simulink model "fancy_dancy_racing_wheely"  (R2019b)
settings: Solver=VariableStepAuto  StartTime=0.0  StopTime=inf  RelTol=1e-3
libraries: dspsrcs4 x2
settings Model: EnablePacing=on  Creator=mandl  LastModifiedBy=mandl

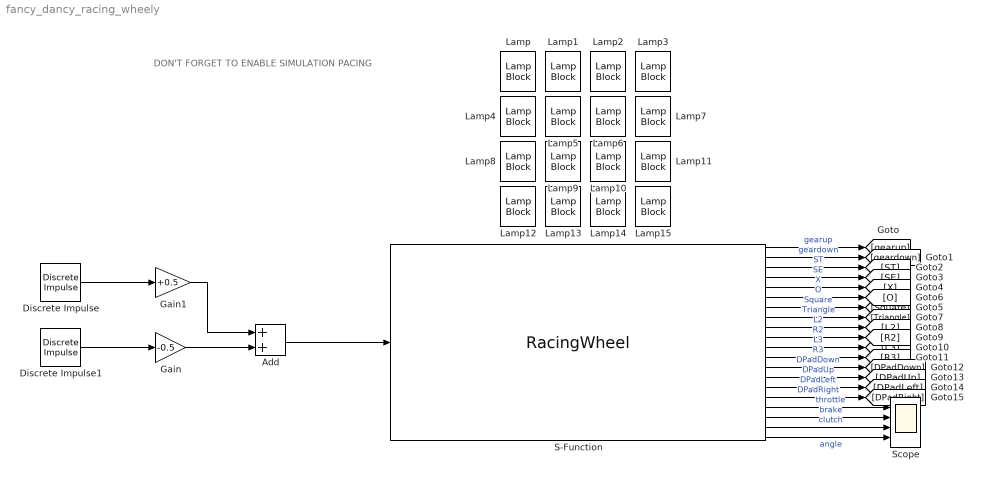
== system fancy_dancy_racing_wheely ==
  note: DON'T FORGET TO ENABLE SIMULATION PACING
  Add : Sum
  Discrete Impulse : dspsrcs4/Discrete  Impulse  Delay=500  SampleTime=0.01  FrameSample=1  OutputFrames=off  dataType=double  isSigned=on  wordLen=16  udDataType=sfix(16)  fracBitsMode=Best precision  numFracBits=15  OutDataTypeStr=double  LastOutDataTypeStr=double
  Discrete Impulse1 : dspsrcs4/Discrete  Impulse  Delay=1000  SampleTime=0.01  FrameSample=1  OutputFrames=off  dataType=double  isSigned=on  wordLen=16  udDataType=sfix(16)  fracBitsMode=Best precision  numFracBits=15  OutDataTypeStr=double  LastOutDataTypeStr=double
  Gain : Gain  Gain=-0.5
  Gain1 : Gain  Gain=+0.5
  Lamp{,1..15} (16 alike) : LampBlock
  S-Function : S-Function  FunctionName=RacingWheel  Parameters=Ts_FF uint32(1e5)  SFunctionModules=RacingWheel_wrapper  SFunctionDeploymentMode=off  EnableBusSupport=off  mask(Racing Wheel with Force Feedback){Ts_FF=0.01, Effect_duration=1e4}
      mask prompts: Ts_FF "Constant Force-Feedback Sample Time"; Effect_duration "Effect Duration in seconds (uint32)"
      mask help: Interacts with the windows gaming API from UWP. The force feedback effect is constant over the user defined sampling time below.
      mask init:
      | val = [[.9  0.75 0.75 1 1 .9 .9 1]',[1 1 0.75 0.75 .9 .9 1 .9]'];try , sys = get_param(gcb,'SfunBuilderFcnName');if isempty(sys), sys = get_param(gcb,'FunctionName'); end,catch, sys = get_param(gcb,'FunctionName'); end
      mask Display:
      | plot(val(:,1),val(:,2)),disp(sys),
      | image('icon.png'),
      | port_label('input',1,'FF'),
      | port_label('output',1,'gearup'),
      | port_label('output',2,'geardown'),
      | port_label('output',3,'ST'),
      | port_label('output',4,'SE'),
      | port_label('output',5,'X'),
      | port_label('output',6,'O'),
      | port_label('output',7,'Square'),
      | port_label('output',8,'Triangle'),
      | port_label('output',9,'L2'),
      | port_label('output',10,'R2'),
      | port_label('output',11,'L3'),
      | port_label('output',12,'R3'),
      | port_label('output',13,'DPadDown'),
      | port_label('output',14,'DPadUp'),
      | port_label('output',15,'DPadLeft'),
      | port_label('output',16,'DPadRight'),
      | port_label('output',17,'throttle'),
      | port_label('output',18,'brake'),
      | port_label('output',19,'clutch'),
      | port_label('output',20,'angle')
  Scope : Scope  NumInputPorts=4
  wires:
  S-Function/20 -> Scope/4  "angle"
  S-Function/19 -> Scope/3  "clutch"
  S-Function/18 -> Scope/2  "brake"
  S-Function/17 -> Scope/1  "throttle"
  S-Function/1 -> [gearup]  "gearup"
  S-Function/2 -> [geardown]  "geardown"
  S-Function/3 -> [ST]  "ST"
  S-Function/4 -> [SE]  "SE"
  S-Function/5 -> [X]  "X"
  S-Function/6 -> [O]  "O"
  S-Function/7 -> [Square]  "Square"
  S-Function/8 -> [Triangle]  "Triangle"
  S-Function/9 -> [L2]  "L2"
  S-Function/10 -> [R2]  "R2"
  S-Function/11 -> [L3]  "L3"
  S-Function/12 -> [R3]  "R3"
  S-Function/13 -> [DPadDown]  "DPadDown"
  S-Function/14 -> [DPadUp]  "DPadUp"
  S-Function/15 -> [DPadLeft]  "DPadLeft"
  S-Function/16 -> [DPadRight]  "DPadRight"
  Discrete Impulse1/1 -> Gain/1
  Add/1 -> S-Function/1
  Gain/1 -> Add/2
  Gain1/1 -> Add/1
  Discrete Impulse/1 -> Gain1/1
